simulink model "sampleModel1803"  (R2023a)
settings: Solver=VariableStepAuto  StartTime=0.0  StopTime=10.0  RelTol=1e-3
libraries: hdlsllib x4, simulink x4
settings Model: Creator=user1  LastModifiedBy=user1

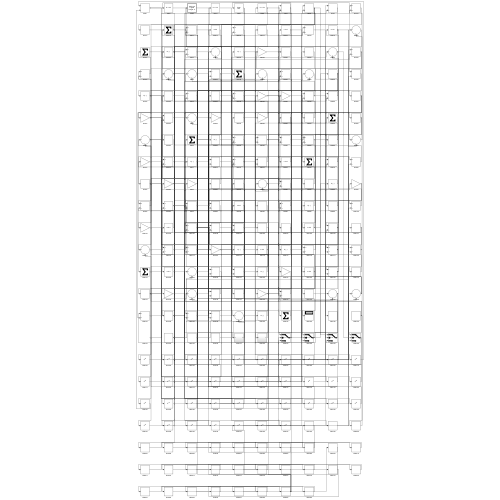
[thumbnail: Simulink's stored preview of the top-level diagram]
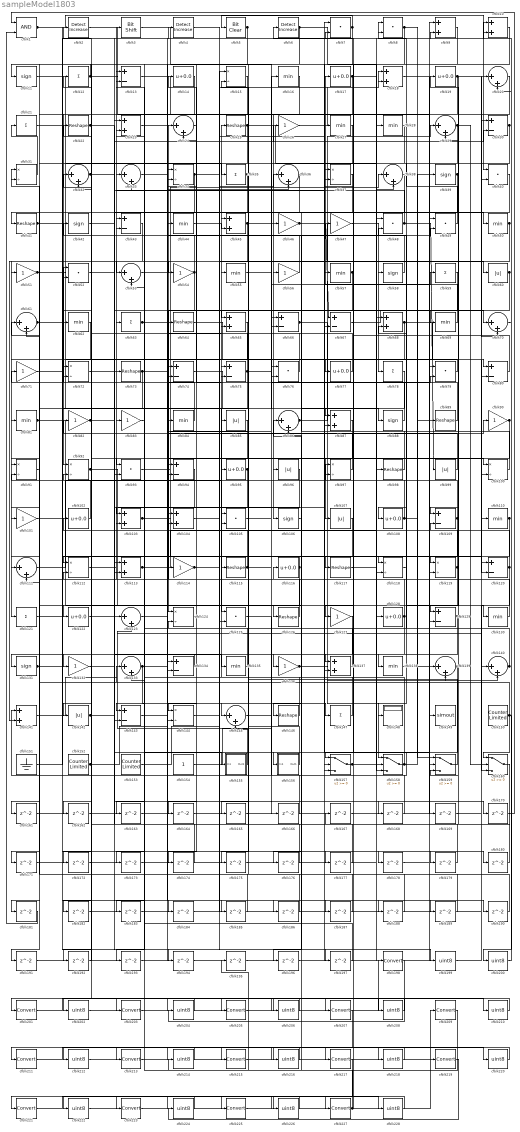
== system sampleModel1803 ==
  cfblk1 : Logic  AllPortsSameDT=off  OutDataTypeStr=boolean
  cfblk{9..10,18,23,45,65,68,87,103..104,113,137,141} (13 alike) : Sum
  cfblk{15,31,34,37,72,91..92,97,100,112,118..119,124,144} (14 alike) : Product  Inputs=*/  RndMeth=Zero  SaturateOnIntegerOverflow=on
  cfblk{26,46..47,51,54,56,71,82..83,90,101,114,127,132,136} (15 alike) : Gain
  cfblk{14,17,19,77,95,102,108,116,122,128} (10 alike) : Bias  Bias=0.0  SaturateOnIntegerOverflow=off
  cfblk{7..8,40,48..49,52,76,79,93,105,125} (11 alike) : DotProduct  OutDataTypeStr=Inherit: Inherit via internal rule
  cfblk{11,39,42,58,88,106,131} (7 alike) : Signum
  cfblk{60,85,96,99,107,142} (6 alike) : Abs  SaturateOnIntegerOverflow=off
  cfblk{13,30,43,66..67,74..75,80,94,109,120,129,134,143} (14 alike) : Sum  Inputs=+-
  cfblk{16,27..28,44,50,55,57,62,69,81,84,110,130,135,138} (15 alike) : MinMax
  cfblk{20,24,29,32..33,36,38,53,61,70,86,111,123,133,139..140,145} (17 alike) : Sum  Inputs=|++
  cfblk{22,25,41,64,73,89,98,115,117,126,146} (11 alike) : Reshape
  cfblk{12,21,35,59,63,78,121,147} (8 alike) : Sum  Inputs=+
  cfblk148 : Display
  cfblk149 : ToWorkspace  VariableName=simout  SaveFormat=Timeseries  SampleTime=-1
  cfblk150 : hdlsllib/Sources/Counter Limited  uplimit=7  tsamp=-1
  cfblk151 : Ground
  cfblk152 : hdlsllib/Sources/Counter Limited  uplimit=7  tsamp=-1
  cfblk153 : hdlsllib/Sources/Counter Limited  uplimit=7  tsamp=-1
  cfblk154 : Constant  SampleTime=-1
  cfblk155 : Subsystem
      settings: LibrarySourceBlock=|
      | hdlsllib/Ports &
      | Subsystems/Subsystem
  cfblk156 : Subsystem
      settings: LibrarySourceBlock=|
      | hdlsllib/Ports &
      | Subsystems/Subsystem
  cfblk{157..160} (4 alike) : Switch  SaturateOnIntegerOverflow=off  InputSameDT=off
  cfblk{161..197} (37 alike) : Delay  SampleTime=1
  cfblk{198,201,203,205,207,209,211,213,215,217,219,221,223,225,227} (15 alike) : DataTypeConversion  SaturateOnIntegerOverflow=off  RndMeth=Floor
  cfblk{199..200,202,204,206,208,210,212,214,216,218,220,222,224,226,228} (16 alike) : DataTypeConversion  OutDataTypeStr=uint8  SaturateOnIntegerOverflow=off  RndMeth=Floor
  cfblk2 : simulink/Logic and Bit Operations/Detect Increase  vinit=0.0  OutDataTypeStr=boolean
      settings: LibrarySourceBlock=|
      | hdlsllib/Logic and Bit
      | Operations/Detect
      | Increase
  cfblk3 : hdlsllib/Logic and Bit Operations/Bit Shift  mode=Shift Left Logical  N=0
  cfblk4 : simulink/Logic and Bit Operations/Detect Increase  vinit=0.0  OutDataTypeStr=boolean
      settings: LibrarySourceBlock=|
      | hdlsllib/Logic and Bit
      | Operations/Detect
      | Increase
  cfblk5 : simulink/Logic and Bit Operations/Bit Clear  iBit=0
      settings: LibrarySourceBlock=|
      | hdlsllib/Logic and Bit
      | Operations/Bit Clear
  cfblk6 : simulink/Logic and Bit Operations/Detect Increase  vinit=0.0  OutDataTypeStr=boolean
      settings: LibrarySourceBlock=|
      | hdlsllib/Logic and Bit
      | Operations/Detect
      | Increase
  wires:
  cfblk54/1 -> cfblk24/1, cfblk144/2
  cfblk81/1 -> cfblk130/1, cfblk4/1
  cfblk57/1 -> cfblk124/1, cfblk86/2
  cfblk2/1 -> cfblk24/2
  cfblk98/1 -> cfblk6/1
  cfblk16/1 -> cfblk92/1
  cfblk97/1 -> cfblk82/1
  cfblk45/1 -> cfblk121/1, cfblk87/2
  cfblk1/1 -> cfblk40/1, cfblk119/2
  cfblk147/1 -> cfblk25/1
  cfblk29/1 -> cfblk118/1, cfblk160/2
  cfblk111/1 -> cfblk55/1
  cfblk31/1 -> cfblk21/1
  cfblk62/1 -> cfblk81/1
  cfblk112/1 -> cfblk3/1
  cfblk158/1 -> cfblk102/1, cfblk39/1
  cfblk75/1 -> cfblk13/1, cfblk79/2, cfblk161/1
  cfblk13/1 -> cfblk106/1
  cfblk133/1 -> cfblk145/1, cfblk7/2
  cfblk102/1 -> cfblk31/1
  cfblk86/1 -> cfblk29/1, cfblk126/1
  cfblk152/1 -> cfblk23/1, cfblk104/2
  cfblk39/1 -> cfblk175/1, cfblk176/1
  cfblk92/1 -> cfblk134/1, cfblk137/2
  cfblk103/1 -> cfblk38/1, cfblk120/2, cfblk129/2, cfblk189/1
  cfblk7/1 -> cfblk5/1, cfblk62/1, cfblk192/1
  cfblk129/1 -> cfblk19/1, cfblk191/1
  cfblk126/1 -> cfblk44/1
  cfblk19/1 -> cfblk109/1, cfblk142/1, cfblk70/2
  cfblk48/1 -> cfblk99/1, cfblk33/2
  cfblk117/1 -> cfblk98/1
  cfblk139/1 -> cfblk141/1, cfblk183/1
  cfblk130/1 -> cfblk43/1
  cfblk4/1 -> cfblk147/1
  cfblk49/1 -> cfblk8/1
  cfblk11/1 -> cfblk125/1
  cfblk137/1 -> cfblk43/2
  cfblk51/1 -> cfblk128/1, cfblk188/1
  cfblk18/1 -> cfblk60/1
  cfblk40/1 -> cfblk53/1
  cfblk96/1 -> cfblk125/2
  cfblk85/1 -> cfblk105/1
  cfblk155/1(Out1) -> cfblk123/2
  cfblk12/1 -> cfblk11/1, cfblk149/1
  cfblk156/1(Out1) -> cfblk84/1
  cfblk142/1 -> cfblk37/1, cfblk190/1
  cfblk150/1 -> cfblk160/1, cfblk92/2, cfblk61/1, cfblk200/1
  cfblk120/1 -> cfblk63/1, cfblk160/3
  cfblk107/1 -> cfblk156/1(In1)
  cfblk24/1 -> cfblk64/1
  cfblk9/1 -> cfblk54/1
  cfblk123/1 -> cfblk75/1
  cfblk134/1 -> cfblk132/1
  cfblk5/1 -> cfblk143/1, cfblk94/2
  cfblk105/1 -> cfblk16/1
  cfblk69/1 -> cfblk17/1
  cfblk41/1 -> cfblk80/1, cfblk87/1
  cfblk47/1 -> cfblk78/1
  cfblk53/1 -> cfblk100/1
  cfblk90/1 -> cfblk119/1, cfblk122/1
  cfblk110/1 -> cfblk109/2, cfblk148/1
  cfblk74/1 -> cfblk88/1
  cfblk154/1 -> cfblk76/1
  cfblk43/1 -> cfblk141/2
  cfblk42/1 -> cfblk155/1(In1)
  cfblk33/1 -> cfblk104/1
  cfblk61/1 -> cfblk186/1, cfblk187/1
  cfblk108/1 -> cfblk83/1, cfblk89/1
  cfblk94/1 -> cfblk103/1
  cfblk119/1 -> cfblk12/1, cfblk138/1
  cfblk89/1 -> cfblk45/1
  cfblk159/1 -> cfblk115/1
  cfblk37/1 -> cfblk93/1
  cfblk8/1 -> cfblk144/1, cfblk127/1, cfblk159/1, cfblk97/2
  cfblk26/1 -> cfblk18/1
  cfblk127/1 -> cfblk143/2
  cfblk91/1 -> cfblk31/2
  cfblk109/1 -> cfblk72/2, cfblk174/1
  cfblk34/1 -> cfblk111/1, cfblk58/1
  cfblk50/1 -> cfblk56/1, cfblk136/1, cfblk93/2
  cfblk113/1 -> cfblk28/1, cfblk49/2
  cfblk143/1 -> cfblk90/1
  cfblk66/1 -> cfblk140/2, cfblk159/2
  cfblk84/1 -> cfblk52/1
  cfblk6/1 -> cfblk145/2, cfblk158/3
  cfblk77/1 -> cfblk14/1
  cfblk88/1 -> cfblk34/2
  cfblk140/1 -> cfblk124/2, cfblk68/2, cfblk97/1
  cfblk44/1 -> cfblk45/2
  cfblk100/1 -> cfblk42/1
  cfblk136/1 -> cfblk158/1, cfblk8/2
  cfblk64/1 -> cfblk76/2
  cfblk72/1 -> cfblk73/1
  cfblk144/1 -> cfblk36/1
  cfblk93/1 -> cfblk46/1
  cfblk28/1 -> cfblk91/1
  cfblk46/1 -> cfblk67/1, cfblk139/1
  cfblk63/1 -> cfblk36/2, cfblk96/1
  cfblk116/1 -> cfblk112/1, cfblk131/1
  cfblk67/1 -> cfblk70/1
  cfblk115/1 -> cfblk59/1, cfblk22/1
  cfblk82/1 -> cfblk184/1, cfblk185/1
  cfblk15/1 -> cfblk41/1
  cfblk17/1 -> cfblk139/2, cfblk182/1
  cfblk83/1 -> cfblk23/2
  cfblk68/1 -> cfblk120/1, cfblk133/2
  cfblk128/1 -> cfblk95/1, cfblk61/2, cfblk171/1, cfblk172/1
  cfblk99/1 -> cfblk85/1
  cfblk56/1 -> cfblk15/2
  cfblk27/1 -> cfblk67/2
  cfblk38/1 -> cfblk51/1
  cfblk106/1 -> cfblk146/1
  cfblk59/1 -> cfblk137/1
  cfblk151/1 -> cfblk72/1
  cfblk141/1 -> cfblk110/1
  cfblk95/1 -> cfblk113/2, cfblk173/1
  cfblk35/1 -> cfblk65/1, cfblk163/1
  cfblk58/1 -> cfblk2/1
  cfblk14/1 -> cfblk74/2
  cfblk114/1 -> cfblk18/2, cfblk180/1
  cfblk76/1 -> cfblk32/1
  cfblk55/1 -> cfblk30/2
  cfblk87/1 -> cfblk107/1
  cfblk32/1 -> cfblk50/1, cfblk26/1
  cfblk146/1 -> cfblk91/2
  cfblk30/1 -> cfblk157/1, cfblk129/1
  cfblk60/1 -> cfblk117/1, cfblk108/1
  cfblk101/1 -> cfblk114/1
  cfblk3/1 -> cfblk66/2
  cfblk79/1 -> cfblk77/1
  cfblk52/1 -> cfblk135/1
  cfblk22/1 -> cfblk10/1, cfblk69/1
  cfblk153/1 -> cfblk27/1
  cfblk135/1 -> cfblk71/1
  cfblk131/1 -> cfblk52/2, cfblk194/1
  cfblk21/1 -> cfblk35/1
  cfblk118/1 -> cfblk48/2
  cfblk80/1 -> cfblk57/1
  cfblk70/1 -> cfblk10/2
  cfblk73/1 -> cfblk65/2, cfblk101/1
  cfblk25/1 -> cfblk158/2, cfblk193/1
  cfblk157/1 -> cfblk9/2, cfblk37/2
  cfblk161/1 -> cfblk123/1
  cfblk65/1 -> cfblk162/1
  cfblk162/1 -> cfblk100/2
  cfblk163/1 -> cfblk13/2
  cfblk124/1 -> cfblk164/1
  cfblk164/1 -> cfblk79/1
  cfblk36/1 -> cfblk165/1
  cfblk165/1 -> cfblk140/1
  cfblk125/1 -> cfblk166/1
  cfblk166/1 -> cfblk66/1
  cfblk160/1 -> cfblk167/1
  cfblk167/1 -> cfblk30/1
  cfblk145/1 -> cfblk168/1
  cfblk168/1 -> cfblk34/1
  cfblk138/1 -> cfblk169/1
  cfblk169/1 -> cfblk29/2
  cfblk122/1 -> cfblk170/1
  cfblk170/1 -> cfblk1/1
  cfblk171/1 -> cfblk48/1
  cfblk172/1 -> cfblk157/2
  cfblk173/1 -> cfblk133/1
  cfblk174/1 -> cfblk113/1
  cfblk175/1 -> cfblk118/2
  cfblk176/1 -> cfblk32/2
  cfblk23/1 -> cfblk177/1
  cfblk177/1 -> cfblk105/2
  cfblk121/1 -> cfblk178/1
  cfblk178/1 -> cfblk49/1
  cfblk71/1 -> cfblk179/1
  cfblk179/1 -> cfblk86/1
  cfblk180/1 -> cfblk159/3
  cfblk10/1 -> cfblk181/1
  cfblk181/1 -> cfblk1/2
  cfblk182/1 -> cfblk15/1
  cfblk183/1 -> cfblk80/2
  cfblk184/1 -> cfblk38/2
  cfblk185/1 -> cfblk94/1
  cfblk186/1 -> cfblk74/1
  cfblk187/1 -> cfblk7/1
  cfblk188/1 -> cfblk75/2
  cfblk189/1 -> cfblk111/2
  cfblk190/1 -> cfblk53/2
  cfblk191/1 -> cfblk68/1
  cfblk192/1 -> cfblk112/2
  cfblk193/1 -> cfblk134/2
  cfblk194/1 -> cfblk157/3
  cfblk195/1 -> cfblk40/2
  cfblk78/1 -> cfblk196/1
  cfblk196/1 -> cfblk9/1
  cfblk104/1 -> cfblk197/1
  cfblk197/1 -> cfblk33/1
  cfblk132/1 -> cfblk199/1
  cfblk199/1 -> cfblk20/1
  cfblk200/1 -> cfblk20/2
  cfblk20/1 -> cfblk202/1
  cfblk202/1 -> cfblk198/1
  cfblk198/1 -> cfblk204/1
  cfblk204/1 -> cfblk201/1
  cfblk201/1 -> cfblk206/1
  cfblk206/1 -> cfblk203/1
  cfblk203/1 -> cfblk208/1
  cfblk208/1 -> cfblk205/1
  cfblk205/1 -> cfblk210/1
  cfblk210/1 -> cfblk207/1
  cfblk207/1 -> cfblk212/1
  cfblk212/1 -> cfblk209/1
  cfblk209/1 -> cfblk214/1
  cfblk214/1 -> cfblk211/1
  cfblk211/1 -> cfblk216/1
  cfblk216/1 -> cfblk213/1
  cfblk213/1 -> cfblk218/1
  cfblk218/1 -> cfblk215/1
  cfblk215/1 -> cfblk220/1
  cfblk220/1 -> cfblk217/1
  cfblk217/1 -> cfblk222/1
  cfblk222/1 -> cfblk219/1
  cfblk219/1 -> cfblk224/1
  cfblk224/1 -> cfblk221/1
  cfblk225/1 -> cfblk227/1
  cfblk221/1 -> cfblk226/1
  cfblk226/1 -> cfblk223/1
  cfblk227/1 -> cfblk195/1, cfblk47/1, cfblk103/2, cfblk116/1
  cfblk223/1 -> cfblk228/1
  cfblk228/1 -> cfblk225/1

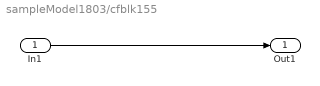
== system sampleModel1803/cfblk155 ==
  In1 : Inport
  Out1 : Outport
  wires:
  In1/1 -> Out1/1

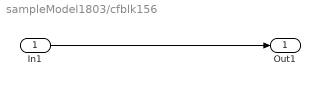
== system sampleModel1803/cfblk156 ==
  In1 : Inport
  Out1 : Outport
  wires:
  In1/1 -> Out1/1
